simulink model "sampler_23b"  (R2023b)
settings: Solver=VariableStepAuto  StartTime=0.0  StopTime=30  RelTol=1e-3
values from neighbouring files (symbols this model uses):
  X = x(:,1)    [UAVs.m]
  xd = cell2mat(Xd)    [UAVs.m]
  Y = x(:,2)    [UAVs.m]
  yd = cell2mat(Yd)    [UAVs.m]
  Z = x(:,3)    [UAVs.m]
  zd = cell2mat(Zd)    [UAVs.m]
settings Model: Creator=bojack  LastModifiedBy=bojack
settings RTWCC: GPUComputeCapability=5.0

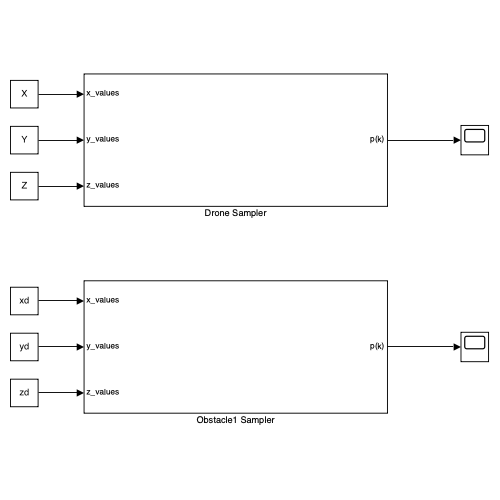
[thumbnail: Simulink's stored preview of the top-level diagram]
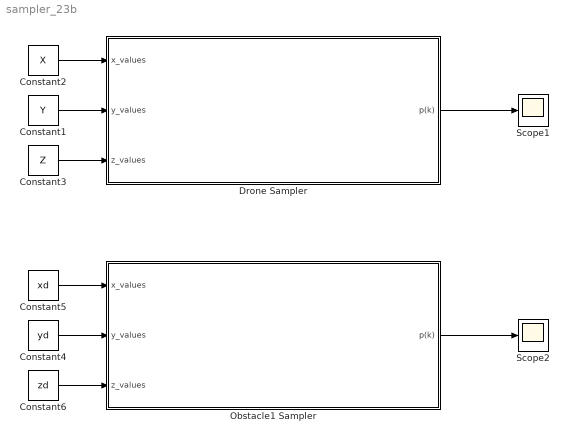
== system sampler_23b ==
  Constant1 : Constant  Value=Y
  Constant2 : Constant  Value=X
  Constant3 : Constant  Value=Z
  Constant4 : Constant  Value=yd
  Constant5 : Constant  Value=xd
  Constant6 : Constant  Value=zd
  Drone Sampler : Subsystem
  Obstacle1 Sampler : Subsystem
  Scope1 : Scope
  Scope2 : Scope
  wires:
  Drone Sampler/1(p(k)) -> Scope1/1
  Constant2/1 -> Drone Sampler/1(x_values)
  Constant1/1 -> Drone Sampler/2(y_values)
  Constant3/1 -> Drone Sampler/3(z_values)
  Constant6/1 -> Obstacle1 Sampler/3(z_values)
  Obstacle1 Sampler/1(p(k)) -> Scope2/1
  Constant5/1 -> Obstacle1 Sampler/1(x_values)
  Constant4/1 -> Obstacle1 Sampler/2(y_values)

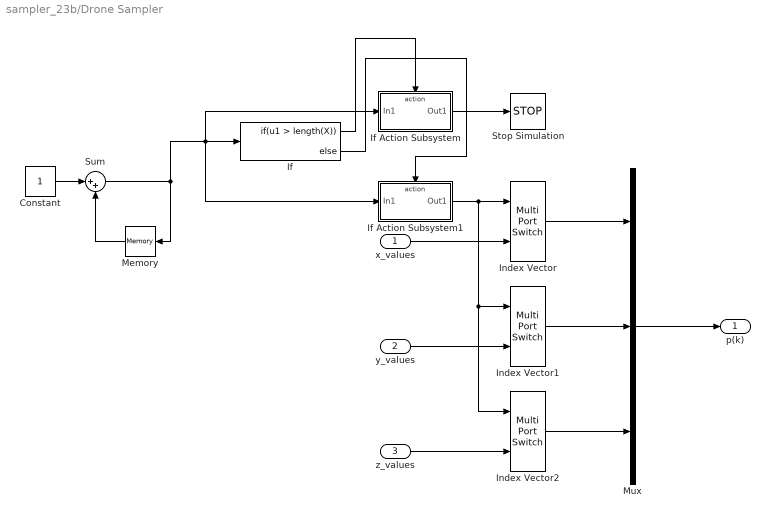
== system sampler_23b/Drone Sampler ==
  x_values : Inport
  y_values : Inport  Port=2
  z_values : Inport  Port=3
  Constant : Constant
  If : If  IfExpression=u1 > length(X)
  If Action Subsystem : Subsystem  TreatAsAtomicUnit=on
  If Action Subsystem1 : Subsystem  TreatAsAtomicUnit=on
  Index Vector : MultiPortSwitch  Inputs=1  SaturateOnIntegerOverflow=off  InputSameDT=off
  Index Vector1 : MultiPortSwitch  Inputs=1  SaturateOnIntegerOverflow=off  InputSameDT=off
  Index Vector2 : MultiPortSwitch  Inputs=1  SaturateOnIntegerOverflow=off  InputSameDT=off
  Memory : Memory
  Mux : Mux  Inputs=3
  Stop Simulation : Stop
  Sum : Sum  Inputs=|++
  p(k) : Outport
  wires:
  x_values/1 -> Index Vector/2
  If Action Subsystem/1(Out1) -> Stop Simulation/1
  If Action Subsystem1/1(Out1) -> Index Vector/1, Index Vector1/1, Index Vector2/1
  If/1 -> If Action Subsystem/Action
  Memory/1 -> Sum/2
  Sum/1 -> If Action Subsystem/1(In1), If/1, If Action Subsystem1/1(In1), Memory/1
  If/2 -> If Action Subsystem1/Action
  Constant/1 -> Sum/1
  y_values/1 -> Index Vector1/2
  z_values/1 -> Index Vector2/2
  Index Vector1/1 -> Mux/2
  Index Vector/1 -> Mux/1
  Index Vector2/1 -> Mux/3
  Mux/1 -> p(k)/1

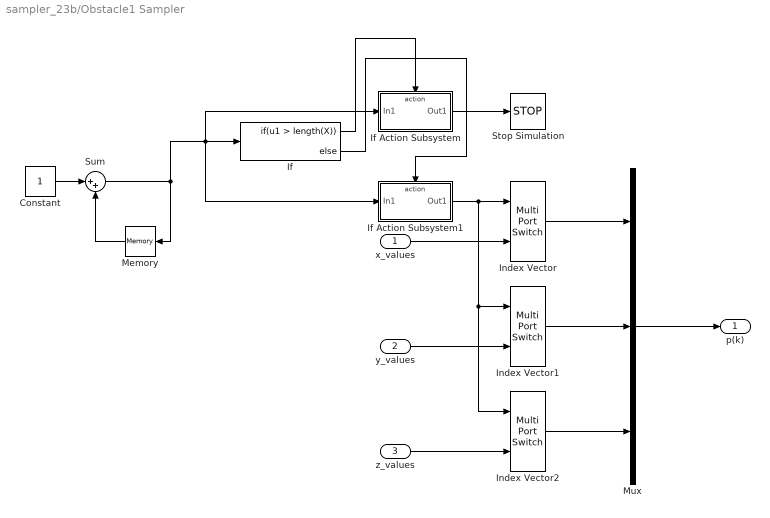
== system sampler_23b/Obstacle1 Sampler ==
  x_values : Inport
  y_values : Inport  Port=2
  z_values : Inport  Port=3
  Constant : Constant
  If : If  IfExpression=u1 > length(X)
  If Action Subsystem : Subsystem  TreatAsAtomicUnit=on
  If Action Subsystem1 : Subsystem  TreatAsAtomicUnit=on
  Index Vector : MultiPortSwitch  Inputs=1  SaturateOnIntegerOverflow=off  InputSameDT=off
  Index Vector1 : MultiPortSwitch  Inputs=1  SaturateOnIntegerOverflow=off  InputSameDT=off
  Index Vector2 : MultiPortSwitch  Inputs=1  SaturateOnIntegerOverflow=off  InputSameDT=off
  Memory : Memory
  Mux : Mux  Inputs=3
  Stop Simulation : Stop
  Sum : Sum  Inputs=|++
  p(k) : Outport
  wires:
  x_values/1 -> Index Vector/2
  If Action Subsystem/1(Out1) -> Stop Simulation/1
  If Action Subsystem1/1(Out1) -> Index Vector/1, Index Vector1/1, Index Vector2/1
  If/1 -> If Action Subsystem/Action
  Memory/1 -> Sum/2
  Sum/1 -> If Action Subsystem/1(In1), If/1, If Action Subsystem1/1(In1), Memory/1
  If/2 -> If Action Subsystem1/Action
  Constant/1 -> Sum/1
  y_values/1 -> Index Vector1/2
  z_values/1 -> Index Vector2/2
  Index Vector1/1 -> Mux/2
  Index Vector/1 -> Mux/1
  Index Vector2/1 -> Mux/3
  Mux/1 -> p(k)/1

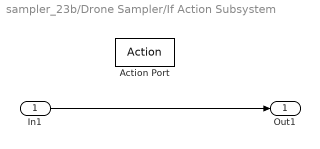
== system sampler_23b/Drone Sampler/If Action Subsystem ==
  In1 : Inport
  Action Port : ActionPort  ActionPortLabel=if(u1 > length(X))
  Out1 : Outport
  wires:
  In1/1 -> Out1/1

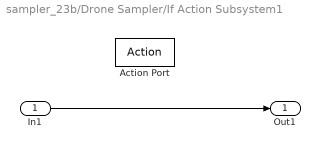
== system sampler_23b/Drone Sampler/If Action Subsystem1 ==
  In1 : Inport
  Action Port : ActionPort  ActionPortLabel=else
  Out1 : Outport
  wires:
  In1/1 -> Out1/1

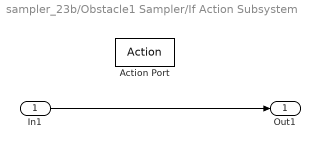
== system sampler_23b/Obstacle1 Sampler/If Action Subsystem ==
  In1 : Inport
  Action Port : ActionPort  ActionPortLabel=if(u1 > length(X))
  Out1 : Outport
  wires:
  In1/1 -> Out1/1

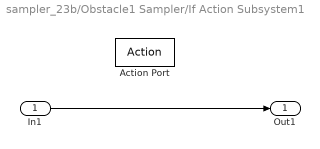
== system sampler_23b/Obstacle1 Sampler/If Action Subsystem1 ==
  In1 : Inport
  Action Port : ActionPort  ActionPortLabel=else
  Out1 : Outport
  wires:
  In1/1 -> Out1/1
